simulink model "Lab3_es4"  (R2024b)
settings: Solver=VariableStepAuto  StartTime=0.0  StopTime=10000  MaxStep=1  RelTol=1e-3
values from neighbouring files (symbols this model uses):
  Gb = 81    [Lab3_param_e_codice.m]
  Ib = 15    [Lab3_param_e_codice.m]
  n = 5/54    (= 0.0925925925926)    [Lab3_param_e_codice.m]
  p1 = P1    (= 0.003)    [Lab3_param_e_codice.m]
  p2 = P2    (= 0.025)    [Lab3_param_e_codice.m]
  p3 = P3    (= 1.3e-05)    [Lab3_param_e_codice.m]
  Ub = 16.66667    [Lab3_param_e_codice.m]
  V1 = 12    [Lab3_param_e_codice.m]
  Vg = 126    [Lab3_param_e_codice.m]
libraries: simulink x4
settings Model: Creator=Diego Regruto  LastModifiedBy=stefa
settings RTWCC: GPUComputeCapability=3.5

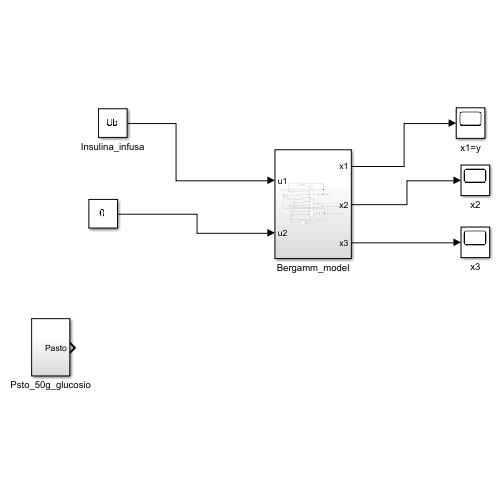
[thumbnail: Simulink's stored preview of the top-level diagram]
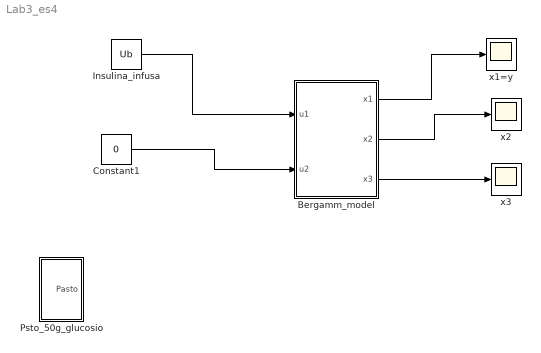
== system Lab3_es4 ==
  Bergamm_model : Subsystem
  Constant1 : Constant  Value=0
  Insulina_infusa : Constant  Value=Ub
  Psto_50g_glucosio : Subsystem
  x1=y : Scope
  x2 : Scope
  x3 : Scope
  wires:
  Insulina_infusa/1 -> Bergamm_model/1(u1)
  Bergamm_model/1(x1) -> x1=y/1
  Bergamm_model/2(x2) -> x2/1
  Bergamm_model/3(x3) -> x3/1
  Constant1/1 -> Bergamm_model/2(u2)

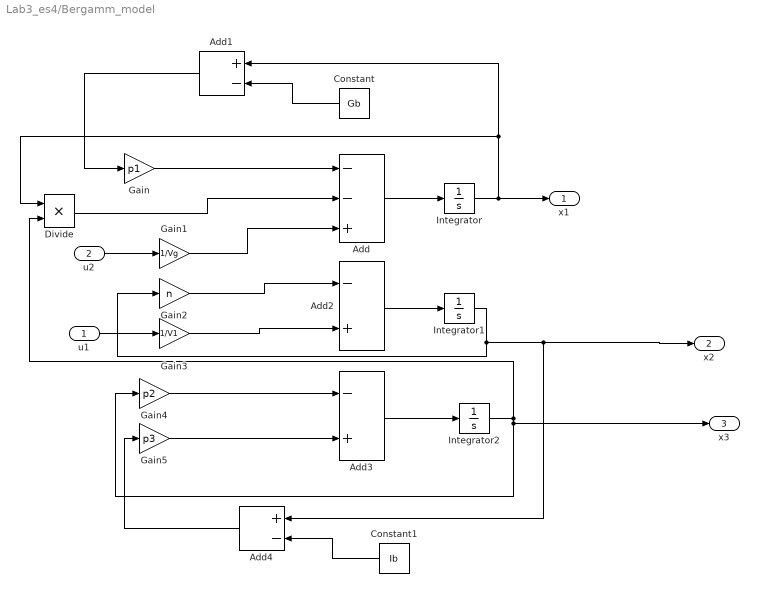
== system Lab3_es4/Bergamm_model ==
  u1 : Inport
  u2 : Inport  Port=2
  Add : Sum  Inputs=--+
  Add1 : Sum  Inputs=+-
  Add2 : Sum  Inputs=-+
  Add3 : Sum  Inputs=-+
  Add4 : Sum  Inputs=+-
  Constant : Constant  Value=Gb
  Constant1 : Constant  Value=Ib
  Divide : Product  Inputs=**
  Gain : Gain  Gain=p1
  Gain1 : Gain  Gain=1/Vg
  Gain2 : Gain  Gain=n
  Gain3 : Gain  Gain=1/V1
  Gain4 : Gain  Gain=p2
  Gain5 : Gain  Gain=p3
  Integrator : Integrator  InitialCondition=81
  Integrator1 : Integrator  InitialCondition=15
  Integrator2 : Integrator
  x1 : Outport
  x2 : Outport  Port=2
  x3 : Outport  Port=3
  wires:
  Constant/1 -> Add1/2
  Add4/1 -> Gain5/1
  Divide/1 -> Add/2
  Integrator1/1 -> x2/1, Add4/1, Gain2/1
  Add3/1 -> Integrator2/1
  Constant1/1 -> Add4/2
  Integrator/1 -> x1/1, Divide/1, Add1/1
  Add/1 -> Integrator/1
  Gain4/1 -> Add3/1
  u2/1 -> Gain1/1
  Gain2/1 -> Add2/1
  u1/1 -> Gain3/1
  Add1/1 -> Gain/1
  Gain/1 -> Add/1
  Add2/1 -> Integrator1/1
  Gain3/1 -> Add2/2
  Integrator2/1 -> Divide/2, x3/1, Gain4/1
  Gain5/1 -> Add3/2
  Gain1/1 -> Add/3

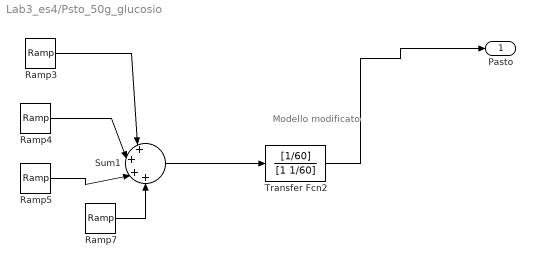
== system Lab3_es4/Psto_50g_glucosio ==
  note: Modello
      | modificato
  Ramp3 : simulink/Sources/Ramp  slope=12  start=0  InitialOutput=0
  Ramp4 : simulink/Sources/Ramp  slope=-12  start=30  InitialOutput=0
  Ramp5 : simulink/Sources/Ramp  slope=-12  start=90  InitialOutput=0
  Ramp7 : simulink/Sources/Ramp  slope=12  start=120  InitialOutput=0
  Sum1 : Sum  Inputs=|+|+|+|+  InputSameDT=on  SaturateOnIntegerOverflow=on  OutDataTypeStr=Inherit: Same as first input
  Transfer Fcn2 : TransferFcn  Numerator=[1/60]  Denominator=[1 1/60]
  Pasto : Outport
  wires:
  Ramp3/1 -> Sum1/1
  Ramp4/1 -> Sum1/2
  Ramp5/1 -> Sum1/3
  Ramp7/1 -> Sum1/4
  Sum1/1 -> Transfer Fcn2/1
  Transfer Fcn2/1 -> Pasto/1
